simulink model "lqr_root_model"  (R2025b)
settings: Solver=VariableStepAuto  StartTime=0.0  StopTime=10.0  RelTol=1e-3
model workspace (MAT data in the model file):
  A = [1  0; 0  1]
  B = [1  0; 0  1]
  C = [1  0; 0  1]
  D = [1  0; 0  1]
  K = [0  0; 0  0]
  body_len = 0.45860001
  body_mass = 1.1
  body_radius = 0.035
  force_gravity = 10.791
  inertia_tensor = Simulink.Parameter
  inertia_tensor.Value = [0.349039299134  0  0; 0  0.349039299134  0; 0  0  0.00067375]
  inertia_tensor.Complexity = 'real'
  inertia_tensor.Dimensions = [3 3]
  inertia_tensor.Description = 'https://en.wikipedia.org/wiki/List_of_moments_of_inertia#List_of_3D_inertia'
  inertia_tensor.DataType = 'auto'
  lever_arm = 0.242
  out = Simulink.SimulationOutput
  out.Data.tout = [0 3.15544362088e-30 3.33352544411e-06 2.00011526647e-05 0.000103339288767 0.000520029969281 0.00260348337185 0.0130207503847 0.0651070854489 0.1 0.159208772587 0.2 ... (2663 elements, 2663x1)]
  out.Metadata = Simulink.SimulationMetadata
  out.Metadata.ModelInfo.ModelName = 'root_model'
  out.Metadata.ModelInfo.ModelVersion = '1.8'
  out.Metadata.ModelInfo.ModelFilePath = 'C:\Users\Josh\Documents\MTU\Involvement\AERE\simulink-testing\mpc-6dof-model\root_model.slx'
  out.Metadata.ModelInfo.UserID = 'Josh'
  out.Metadata.ModelInfo.MachineName = 'DESKTOP-E2GQ9U1'
  out.Metadata.ModelInfo.Platform = 'PCWIN64'
  out.Metadata.ModelInfo.ModelStructuralChecksum = [3232016487; 973311862; 3022833271; 3161490746]
  out.Metadata.ModelInfo.SimulationMode = 'normal'
  out.Metadata.ModelInfo.StartTime = 0
  out.Metadata.ModelInfo.StopTime = 10
  out.Metadata.ModelInfo.SolverInfo.Type = 'Variable-Step'
  out.Metadata.ModelInfo.SolverInfo.Solver = 'ode45'
  out.Metadata.ModelInfo.SolverInfo.MaxStepSize = 0.1
  out.Metadata.ModelInfo.SimulinkVersion.Name = 'Simulink'
  out.Metadata.ModelInfo.SimulinkVersion.Version = '25.2'
  out.Metadata.ModelInfo.SimulinkVersion.Release = '(R2025b)'
  out.Metadata.ModelInfo.SimulinkVersion.Date = '28-Jul-2025'
  out.Metadata.ModelInfo.LoggingInfo.LoggingToFile = 'off'
  out.Metadata.TimingInfo.WallClockTimestampStart = '2026-04-01 21:49:39'
  out.Metadata.TimingInfo.WallClockTimestampStop = '2026-04-01 21:49:46'
  out.Metadata.TimingInfo.InitializationElapsedWallTime = 0.363943
  out.Metadata.TimingInfo.ExecutionElapsedWallTime = 6.470538
  out.Metadata.TimingInfo.TerminationElapsedWallTime = 0.0036556
  out.Metadata.TimingInfo.TotalElapsedWallTime = 6.8381366
  out.Metadata.TimingInfo.ProfilerData = 'Profiler is not enabled'
  out.Metadata.ExecutionInfo.StopEvent = 'ReachedStopTime'
  out.Metadata.ExecutionInfo.StopEventSource = []
  out.Metadata.ExecutionInfo.StopEventDescription = 'Reached stop time of 10'
  out.Metadata.ExecutionInfo.ErrorDiagnostic = []
  out.Metadata.ExecutionInfo.WarningDiagnostics = struct([])
  out.Metadata.AppInfo = struct()
  prop_const = 0.0005967898212
libraries: aerolibanim x1
settings Model: Creator=James  LastModifiedBy=James

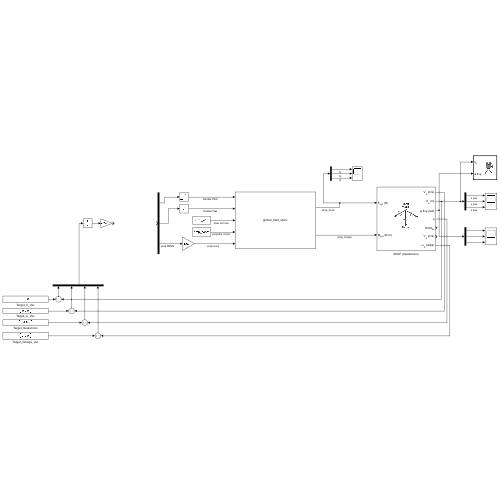
[thumbnail: Simulink's stored preview of the top-level diagram]
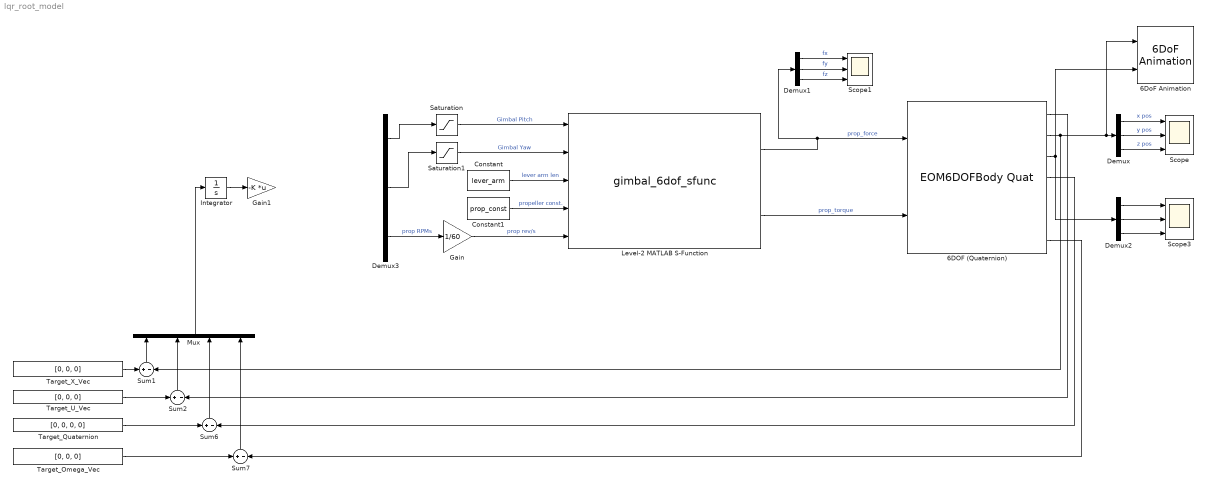
== system lqr_root_model ==
  6DOF (Quaternion) : EOM6DOFBodyQuat  mass_0=body_mass  inertia=inertia_tensor
  6DoF Animation : aerolibanim/6DoF Animation  u1=[0 4000 -2000 2000 -5000 -3000]  u2=0.1  u3=1.0  u4=[4000 0 -5000]  u5=Fly alongside  u6=[2000 500 -3150]  u7=10  u8=on
  Constant : Constant  Value=lever_arm
  Constant1 : Constant  Value=prop_const
  Demux{,1..3} (4 alike) : Demux  Outputs=3
  Gain : Gain  Gain=1/60
  Gain1 : Gain  Gain=-K  Multiplication=Matrix(K*u)
  Integrator : Integrator
  Level-2 MATLAB S-Function : M-S-Function  FunctionName=gimbal_6dof_sfunc
  Mux : Mux
  Saturation : Saturate  UpperLimit=pi  LowerLimit=-pi
  Saturation1 : Saturate  UpperLimit=pi  LowerLimit=-pi
  Scope : Scope  NumInputPorts=3
      settings: ActiveDisplayYMinimum=-1053.7991388199948  ActiveDisplayYMaximum=1498.6999361906014
  Scope1 : Scope  NumInputPorts=3
      settings: ActiveDisplayYMinimum=4.29292633197872  ActiveDisplayYMaximum=72.484649474443529
  Scope3 : Scope  NumInputPorts=3
      settings: ActiveDisplayYMinimum=-0.39668945114680487  ActiveDisplayYMaximum=2.2921731570527948  DataLoggingVariableName=ScopeData3
  Sum{1..2,6..7} (4 alike) : Sum  Inputs=+|-
  Target_Omega_Vec : Constant  Value=[0, 0, 0]
  Target_Quaternion : Constant  Value=[0, 0, 0, 0]
  Target_U_Vec : Constant  Value=[0, 0, 0]
  Target_X_Vec : Constant  Value=[0, 0, 0]
  wires:
  Saturation1/1 -> Level-2 MATLAB S-Function/2  "Gimbal Yaw"
  Demux/2 -> Scope/2  "y pos"
  Demux/1 -> Scope/1  "x pos"
  Demux2/3 -> Scope3/3
  6DOF (Quaternion)/3 -> 6DoF Animation/2, Demux2/1
  Demux1/3 -> Scope1/3  "fz"
  Demux1/2 -> Scope1/2  "fy"
  Constant1/1 -> Level-2 MATLAB S-Function/4  "propeller const."
  Demux2/2 -> Scope3/2
  Level-2 MATLAB S-Function/2 -> 6DOF (Quaternion)/2  "prop_torque"
  Demux3/3 -> Gain/1  "prop RPMs"
  Level-2 MATLAB S-Function/1 -> Demux1/1, 6DOF (Quaternion)/1  "prop_force"
  Demux1/1 -> Scope1/1  "fx"
  Demux/3 -> Scope/3  "z pos"
  Demux2/1 -> Scope3/1
  Constant/1 -> Level-2 MATLAB S-Function/3  "lever arm len"
  Gain/1 -> Level-2 MATLAB S-Function/5  "prop rev/s"
  6DOF (Quaternion)/2 -> Sum1/2, 6DoF Animation/1, Demux/1
  Saturation/1 -> Level-2 MATLAB S-Function/1  "Gimbal Pitch"
  Mux/1 -> Integrator/1
  Demux3/1 -> Saturation/1
  Demux3/2 -> Saturation1/1
  Integrator/1 -> Gain1/1
  6DOF (Quaternion)/1 -> Sum2/2
  6DOF (Quaternion)/4 -> Sum6/2
  6DOF (Quaternion)/7 -> Sum7/2
  Target_X_Vec/1 -> Sum1/1
  Target_U_Vec/1 -> Sum2/1
  Target_Quaternion/1 -> Sum6/1
  Target_Omega_Vec/1 -> Sum7/1
  Sum1/1 -> Mux/1
  Sum2/1 -> Mux/2
  Sum6/1 -> Mux/3
  Sum7/1 -> Mux/4
